simulink model "test_junk"  (Simulink 6.2)
settings: Solver=ode45  StartTime=0.0  StopTime=10.0  RelTol=1e-3
libraries: xbsIndex_r3 x670
(part 3 of 5)

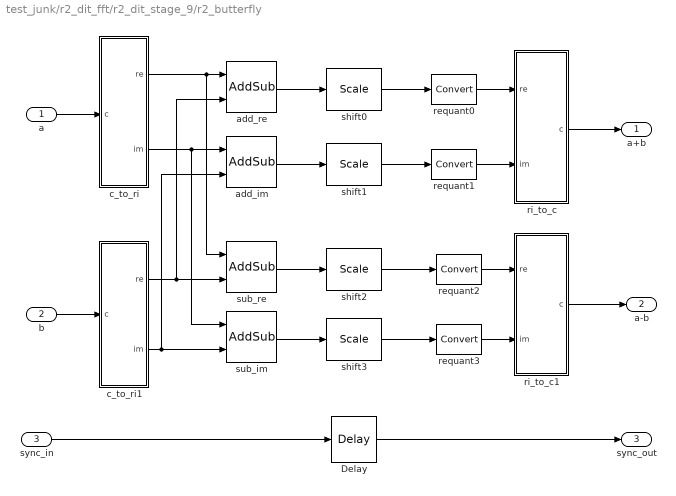
== system test_junk/r2_dit_fft/r2_dit_stage_9/r2_butterfly ==
  a : Inport  Port=1  LatchInput=off
  b : Inport  Port=2  LatchInput=off
  sync_in : Inport  Port=3  LatchInput=off
  Delay : xbsIndex_r3/Delay  latency=1  reg_retiming=off  explicit_period=off  period=1  en=off  accept_only_valid=off  init_zero=on  dbl_ovrd=off  show_param=off
      settings: xl_area=[0, 0, 0, 0, 0, 0, 0]
  add_im : xbsIndex_r3/AddSub  mode=Addition  precision=Full  arith_type=Unsigned  n_bits=8  bin_pt=2  quantization=Truncate  overflow=Wrap  latency=1  explicit_period=off  period=1  use_carryin=off  use_carryout=off  en=off  dbl_ovrd=off  show_param=on  use_core=on  pipeline=on  use_rpm=on  gen_core=off
      settings: xl_area=[0, 0, 0, 0, 0, 0, 0]
  add_re : xbsIndex_r3/AddSub  mode=Addition  precision=Full  arith_type=Unsigned  n_bits=8  bin_pt=2  quantization=Truncate  overflow=Wrap  latency=1  explicit_period=off  period=1  use_carryin=off  use_carryout=off  en=off  dbl_ovrd=off  show_param=on  use_core=on  pipeline=on  use_rpm=on  gen_core=off
      settings: xl_area=[0, 0, 0, 0, 0, 0, 0]
  c_to_ri : Subsystem
      settings: AttributesFormatString=16_0 r/i
  c_to_ri1 : Subsystem
      settings: AttributesFormatString=16_0 r/i
  requant{0..3} (4 alike) : xbsIndex_r3/Convert  arith_type="Signed  (2's comp)"  n_bits=17  bin_pt=0  quantization=Truncate  overflow=Wrap  latency=0  explicit_period=off  period=1  dbl_ovrd=off  show_param=on  inserted_by_tool=off  pipeline=on
      settings: xl_area=[0, 0, 0, 0, 0, 0, 0]
  ri_to_c : Subsystem
  ri_to_c1 : Subsystem
  shift{0..3} (4 alike) : xbsIndex_r3/Scale  scale_factor=0  explicit_period=off  period=1  dbl_ovrd=off
  sub_im : xbsIndex_r3/AddSub  mode=Subtraction  precision=Full  arith_type=Unsigned  n_bits=8  bin_pt=2  quantization=Truncate  overflow=Wrap  latency=1  explicit_period=off  period=1  use_carryin=off  use_carryout=off  en=off  dbl_ovrd=off  show_param=on  use_core=on  pipeline=on  use_rpm=on  gen_core=off
      settings: xl_area=[0, 0, 0, 0, 0, 0, 0]
  sub_re : xbsIndex_r3/AddSub  mode=Subtraction  precision=Full  arith_type=Unsigned  n_bits=8  bin_pt=2  quantization=Truncate  overflow=Wrap  latency=1  explicit_period=off  period=1  use_carryin=off  use_carryout=off  en=off  dbl_ovrd=off  show_param=on  use_core=on  pipeline=on  use_rpm=on  gen_core=off
      settings: xl_area=[0, 0, 0, 0, 0, 0, 0]
  a+b : Outport
  a-b : Outport  Port=2
  sync_out : Outport  Port=3
  wires:
  shift3/1 -> requant3/1
  sub_im/1 -> shift3/1
  shift2/1 -> requant2/1
  sub_re/1 -> shift2/1
  shift1/1 -> requant1/1
  shift0/1 -> requant0/1
  requant3/1 -> ri_to_c1/2(im)
  requant2/1 -> ri_to_c1/1(re)
  requant1/1 -> ri_to_c/2(im)
  requant0/1 -> ri_to_c/1(re)
  Delay/1 -> sync_out/1
  sync_in/1 -> Delay/1
  ri_to_c1/1(c) -> a-b/1
  ri_to_c/1(c) -> a+b/1
  add_im/1 -> shift1/1
  add_re/1 -> shift0/1
  a/1 -> c_to_ri/1(c)
  c_to_ri/2(im) -> sub_im/1, add_im/1
  c_to_ri/1(re) -> sub_re/1, add_re/1
  c_to_ri1/2(im) -> add_im/2, sub_im/2
  c_to_ri1/1(re) -> add_re/2, sub_re/2
  b/1 -> c_to_ri1/1(c)

== system test_junk/r2_dit_fft/r2_dit_stage_9/r2_twiddle ==
  a_in : Inport  Port=1  LatchInput=off
  b : Inport  Port=2  LatchInput=off
  sync_in : Inport  Port=3  LatchInput=off
  Delay1 : xbsIndex_r3/Delay  latency=1  reg_retiming=off  explicit_period=off  period=1  en=off  accept_only_valid=off  init_zero=on  dbl_ovrd=off  show_param=off
      settings: xl_area=[0, 0, 0, 0, 0, 0, 0]
  Delay2 : xbsIndex_r3/Delay  latency=1  reg_retiming=off  explicit_period=off  period=1  en=off  accept_only_valid=off  init_zero=on  dbl_ovrd=off  show_param=off
      settings: xl_area=[0, 0, 0, 0, 0, 0, 0]
  Delay3 : xbsIndex_r3/Delay  latency=1  reg_retiming=off  explicit_period=off  period=1  en=off  accept_only_valid=off  init_zero=on  dbl_ovrd=off  show_param=off
      settings: xl_area=[0, 0, 0, 0, 0, 0, 0]
  cmpy1 : Subsystem
      settings: AttributesFormatString=|
      | 16_15 * 9_7 ==> 16_15
      | round even, wrap
      | 3 mults
  twiddle_gen1 : Subsystem
      settings: AttributesFormatString=|
      | depth 256
      | twiddle bram
  a_out : Outport
  bw : Outport  Port=2
  sync_out : Outport  Port=3
  wires:
  Delay3/1 -> cmpy1/4(sync_in)
  cmpy1/3(sync_out) -> sync_out/1
  twiddle_gen1/1(w) -> cmpy1/3(w)
  cmpy1/2(bw) -> bw/1
  Delay1/1 -> cmpy1/2(b)
  cmpy1/1(a_out) -> a_out/1
  Delay2/1 -> cmpy1/1(a_in)
  a_in/1 -> Delay2/1
  b/1 -> Delay1/1
  sync_in/1 -> Delay3/1, twiddle_gen1/1(sync_in)

== system test_junk/r2_dit_fft/r2_dit_stage_1/biplex_commutator/delay_b ==
  in : Inport  Port=1  LatchInput=off
  Constant : xbsIndex_r3/Constant  const=1  equ=P=C  arith_type=Boolean  n_bits=1  bin_pt=0  opselect=C  inp2=PCIN>>17  opr=+  inp1=P  carry=CIN  iostate=0  explicit_period=on  period=1  dbl_ovrd=off
  Counter : xbsIndex_r3/Counter  cnt_type=Count Limited  n_bits=9  bin_pt=0  arith_type=Unsigned  start_count=0  cnt_to=510  cnt_by_val=1  operation=Up  explicit_period=off  period=1  load_pin=off  rst=off  en=off  dbl_ovrd=off  show_param=off  use_rpm=on  gen_core=off
      settings: xl_area=[0, 0, 0, 0, 0, 0, 0]
  bram : xbsIndex_r3/Single Port RAM  depth=512  initVector=0  write_mode=Read Before Write  latency=1  init_zero=on  explicit_period=off  period=1  rst=off  init_reg=0  en=off  dbl_ovrd=off  show_param=off  distributed_mem=off  use_rpm=off  gen_core=off
      settings: xl_area=[0, 0, 0, 0, 0, 0, 0]
  out : Outport
  wires:
  Constant/1 -> bram/3
  in/1 -> bram/2
  bram/1 -> out/1
  Counter/1 -> bram/1

== system test_junk/r2_dit_fft/r2_dit_stage_1/biplex_commutator/delay_lo ==
  in : Inport  Port=1  LatchInput=off
  Constant : xbsIndex_r3/Constant  const=1  equ=P=C  arith_type=Boolean  n_bits=1  bin_pt=0  opselect=C  inp2=PCIN>>17  opr=+  inp1=P  carry=CIN  iostate=0  explicit_period=on  period=1  dbl_ovrd=off
  Counter : xbsIndex_r3/Counter  cnt_type=Count Limited  n_bits=9  bin_pt=0  arith_type=Unsigned  start_count=0  cnt_to=510  cnt_by_val=1  operation=Up  explicit_period=off  period=1  load_pin=off  rst=off  en=off  dbl_ovrd=off  show_param=off  use_rpm=on  gen_core=off
      settings: xl_area=[0, 0, 0, 0, 0, 0, 0]
  bram : xbsIndex_r3/Single Port RAM  depth=512  initVector=0  write_mode=Read Before Write  latency=1  init_zero=on  explicit_period=off  period=1  rst=off  init_reg=0  en=off  dbl_ovrd=off  show_param=off  distributed_mem=off  use_rpm=off  gen_core=off
      settings: xl_area=[0, 0, 0, 0, 0, 0, 0]
  out : Outport
  wires:
  Constant/1 -> bram/3
  in/1 -> bram/2
  bram/1 -> out/1
  Counter/1 -> bram/1

== system test_junk/r2_dit_fft/r2_dit_stage_1/r2_butterfly/c_to_ri ==
  c : Inport  Port=1  LatchInput=off
  force_im : xbsIndex_r3/Reinterpret  force_arith_type=on  arith_type="Signed  (2's comp)"  force_bin_pt=on  bin_pt=0  force_valid=on
  force_re : xbsIndex_r3/Reinterpret  force_arith_type=on  arith_type="Signed  (2's comp)"  force_bin_pt=on  bin_pt=0  force_valid=on
  slice_im : xbsIndex_r3/Slice  mode=Lower Bit Location + Width  nbits=8  bit1=0  base1=MSB of Input  bit0=0  base0=LSB of Input  boolean_output=off  explicit_period=off  period=1  dbl_ovrd=off
  slice_re : xbsIndex_r3/Slice  mode=Upper Bit Location + Width  nbits=8  bit1=0  base1=MSB of Input  bit0=0  base0=LSB of Input  boolean_output=off  explicit_period=off  period=1  dbl_ovrd=off
  re : Outport
  im : Outport  Port=2
  wires:
  slice_re/1 -> force_re/1
  slice_im/1 -> force_im/1
  force_re/1 -> re/1
  force_im/1 -> im/1
  c/1 -> slice_re/1, slice_im/1

== system test_junk/r2_dit_fft/r2_dit_stage_1/r2_butterfly/c_to_ri1 ==
  c : Inport  Port=1  LatchInput=off
  force_im : xbsIndex_r3/Reinterpret  force_arith_type=on  arith_type="Signed  (2's comp)"  force_bin_pt=on  bin_pt=0  force_valid=on
  force_re : xbsIndex_r3/Reinterpret  force_arith_type=on  arith_type="Signed  (2's comp)"  force_bin_pt=on  bin_pt=0  force_valid=on
  slice_im : xbsIndex_r3/Slice  mode=Lower Bit Location + Width  nbits=8  bit1=0  base1=MSB of Input  bit0=0  base0=LSB of Input  boolean_output=off  explicit_period=off  period=1  dbl_ovrd=off
  slice_re : xbsIndex_r3/Slice  mode=Upper Bit Location + Width  nbits=8  bit1=0  base1=MSB of Input  bit0=0  base0=LSB of Input  boolean_output=off  explicit_period=off  period=1  dbl_ovrd=off
  re : Outport
  im : Outport  Port=2
  wires:
  slice_re/1 -> force_re/1
  slice_im/1 -> force_im/1
  force_re/1 -> re/1
  force_im/1 -> im/1
  c/1 -> slice_re/1, slice_im/1

== system test_junk/r2_dit_fft/r2_dit_stage_1/r2_butterfly/ri_to_c ==
  re : Inport  Port=1  LatchInput=off
  im : Inport  Port=2  LatchInput=off
  concat : xbsIndex_r3/Concat  num_inputs=2  explicit_period=off  period=1  dbl_ovrd=off
  force_im : xbsIndex_r3/Reinterpret  force_arith_type=on  arith_type=Unsigned  force_bin_pt=on  bin_pt=0  force_valid=on
  force_re : xbsIndex_r3/Reinterpret  force_arith_type=on  arith_type=Unsigned  force_bin_pt=on  bin_pt=0  force_valid=on
  c : Outport
  wires:
  force_re/1 -> concat/1
  force_im/1 -> concat/2
  re/1 -> force_re/1
  concat/1 -> c/1
  im/1 -> force_im/1

== system test_junk/r2_dit_fft/r2_dit_stage_1/r2_butterfly/ri_to_c1 ==
  re : Inport  Port=1  LatchInput=off
  im : Inport  Port=2  LatchInput=off
  concat : xbsIndex_r3/Concat  num_inputs=2  explicit_period=off  period=1  dbl_ovrd=off
  force_im : xbsIndex_r3/Reinterpret  force_arith_type=on  arith_type=Unsigned  force_bin_pt=on  bin_pt=0  force_valid=on
  force_re : xbsIndex_r3/Reinterpret  force_arith_type=on  arith_type=Unsigned  force_bin_pt=on  bin_pt=0  force_valid=on
  c : Outport
  wires:
  force_re/1 -> concat/1
  force_im/1 -> concat/2
  re/1 -> force_re/1
  concat/1 -> c/1
  im/1 -> force_im/1

== system test_junk/r2_dit_fft/r2_dit_stage_10/biplex_commutator/delay_b ==
  in : Inport  Port=1  LatchInput=off
  slr : xbsIndex_r3/Delay  latency=1  reg_retiming=off  explicit_period=off  period=1  en=off  accept_only_valid=off  init_zero=on  dbl_ovrd=off  show_param=off
      settings: xl_area=[0, 0, 0, 0, 0, 0, 0]
  out : Outport
  wires:
  slr/1 -> out/1
  in/1 -> slr/1

== system test_junk/r2_dit_fft/r2_dit_stage_10/biplex_commutator/delay_lo ==
  in : Inport  Port=1  LatchInput=off
  slr : xbsIndex_r3/Delay  latency=1  reg_retiming=off  explicit_period=off  period=1  en=off  accept_only_valid=off  init_zero=on  dbl_ovrd=off  show_param=off
      settings: xl_area=[0, 0, 0, 0, 0, 0, 0]
  out : Outport
  wires:
  slr/1 -> out/1
  in/1 -> slr/1

== system test_junk/r2_dit_fft/r2_dit_stage_10/r2_butterfly/c_to_ri ==
  c : Inport  Port=1  LatchInput=off
  force_im : xbsIndex_r3/Reinterpret  force_arith_type=on  arith_type="Signed  (2's comp)"  force_bin_pt=on  bin_pt=0  force_valid=on
  force_re : xbsIndex_r3/Reinterpret  force_arith_type=on  arith_type="Signed  (2's comp)"  force_bin_pt=on  bin_pt=0  force_valid=on
  slice_im : xbsIndex_r3/Slice  mode=Lower Bit Location + Width  nbits=17  bit1=0  base1=MSB of Input  bit0=0  base0=LSB of Input  boolean_output=off  explicit_period=off  period=1  dbl_ovrd=off
  slice_re : xbsIndex_r3/Slice  mode=Upper Bit Location + Width  nbits=17  bit1=0  base1=MSB of Input  bit0=0  base0=LSB of Input  boolean_output=off  explicit_period=off  period=1  dbl_ovrd=off
  re : Outport
  im : Outport  Port=2
  wires:
  slice_re/1 -> force_re/1
  slice_im/1 -> force_im/1
  force_re/1 -> re/1
  force_im/1 -> im/1
  c/1 -> slice_re/1, slice_im/1

== system test_junk/r2_dit_fft/r2_dit_stage_10/r2_butterfly/c_to_ri1 ==
  c : Inport  Port=1  LatchInput=off
  force_im : xbsIndex_r3/Reinterpret  force_arith_type=on  arith_type="Signed  (2's comp)"  force_bin_pt=on  bin_pt=0  force_valid=on
  force_re : xbsIndex_r3/Reinterpret  force_arith_type=on  arith_type="Signed  (2's comp)"  force_bin_pt=on  bin_pt=0  force_valid=on
  slice_im : xbsIndex_r3/Slice  mode=Lower Bit Location + Width  nbits=17  bit1=0  base1=MSB of Input  bit0=0  base0=LSB of Input  boolean_output=off  explicit_period=off  period=1  dbl_ovrd=off
  slice_re : xbsIndex_r3/Slice  mode=Upper Bit Location + Width  nbits=17  bit1=0  base1=MSB of Input  bit0=0  base0=LSB of Input  boolean_output=off  explicit_period=off  period=1  dbl_ovrd=off
  re : Outport
  im : Outport  Port=2
  wires:
  slice_re/1 -> force_re/1
  slice_im/1 -> force_im/1
  force_re/1 -> re/1
  force_im/1 -> im/1
  c/1 -> slice_re/1, slice_im/1

== system test_junk/r2_dit_fft/r2_dit_stage_10/r2_butterfly/ri_to_c ==
  re : Inport  Port=1  LatchInput=off
  im : Inport  Port=2  LatchInput=off
  concat : xbsIndex_r3/Concat  num_inputs=2  explicit_period=off  period=1  dbl_ovrd=off
  force_im : xbsIndex_r3/Reinterpret  force_arith_type=on  arith_type=Unsigned  force_bin_pt=on  bin_pt=0  force_valid=on
  force_re : xbsIndex_r3/Reinterpret  force_arith_type=on  arith_type=Unsigned  force_bin_pt=on  bin_pt=0  force_valid=on
  c : Outport
  wires:
  force_re/1 -> concat/1
  force_im/1 -> concat/2
  re/1 -> force_re/1
  concat/1 -> c/1
  im/1 -> force_im/1

== system test_junk/r2_dit_fft/r2_dit_stage_10/r2_butterfly/ri_to_c1 ==
  re : Inport  Port=1  LatchInput=off
  im : Inport  Port=2  LatchInput=off
  concat : xbsIndex_r3/Concat  num_inputs=2  explicit_period=off  period=1  dbl_ovrd=off
  force_im : xbsIndex_r3/Reinterpret  force_arith_type=on  arith_type=Unsigned  force_bin_pt=on  bin_pt=0  force_valid=on
  force_re : xbsIndex_r3/Reinterpret  force_arith_type=on  arith_type=Unsigned  force_bin_pt=on  bin_pt=0  force_valid=on
  c : Outport
  wires:
  force_re/1 -> concat/1
  force_im/1 -> concat/2
  re/1 -> force_re/1
  concat/1 -> c/1
  im/1 -> force_im/1

== system test_junk/r2_dit_fft/r2_dit_stage_10/r2_twiddle/cmpy1 ==
  a_in : Inport  Port=1  LatchInput=off
  b : Inport  Port=2  LatchInput=off
  w : Inport  Port=3  LatchInput=off
  sync_in : Inport  Port=4  LatchInput=off
  Delay : xbsIndex_r3/Delay  latency=8  reg_retiming=off  explicit_period=off  period=1  en=off  accept_only_valid=off  init_zero=on  dbl_ovrd=off  show_param=off
      settings: xl_area=[1 1 0 1 0 0 0]
  Delay1 : xbsIndex_r3/Delay  latency=8  reg_retiming=off  explicit_period=off  period=1  en=off  accept_only_valid=off  init_zero=on  dbl_ovrd=off  show_param=off
      settings: xl_area=[17 34 0 34 0 0 0]
  br_add_bi : xbsIndex_r3/AddSub  mode=Addition  precision=Full  arith_type=Unsigned  n_bits=8  bin_pt=2  quantization=Truncate  overflow=Wrap  latency=1  explicit_period=off  period=1  use_carryin=off  use_carryout=off  en=off  dbl_ovrd=off  show_param=on  use_core=on  pipeline=on  use_rpm=on  gen_core=off
      settings: xl_area=[9 18 0 18 0 0 0]
  c_to_ri : Subsystem
      settings: AttributesFormatString=17_16 r/i
  c_to_ri1 : Subsystem
      settings: AttributesFormatString=9_7 r/i
  convert_im : xbsIndex_r3/Convert  arith_type="Signed  (2's comp)"  n_bits=17  bin_pt=16  quantization="Round  (unbiased: Even Values)"  overflow=Wrap  latency=3  explicit_period=off  period=1  dbl_ovrd=off  show_param=on  inserted_by_tool=off  pipeline=on
      settings: xl_area=[0, 0, 0, 0, 0, 0, 0]
  convert_re : xbsIndex_r3/Convert  arith_type="Signed  (2's comp)"  n_bits=17  bin_pt=16  quantization="Round  (unbiased: Even Values)"  overflow=Wrap  latency=3  explicit_period=off  period=1  dbl_ovrd=off  show_param=on  inserted_by_tool=off  pipeline=on
      settings: xl_area=[0, 0, 0, 0, 0, 0, 0]
  imim : xbsIndex_r3/Mult  precision=User Defined  arith_type="Signed  (2's comp)"  n_bits=24  bin_pt=23  quantization=Truncate  overflow=Wrap  latency=3  explicit_period=off  period=1  en=off  dbl_ovrd=off  show_param=on  mult_type=Parallel  oversample=2  use_embedded=on  pipeline=on  use_rpm=on  placement_style=Rectangular Shape  gen_core=off
      settings: xl_area=[26 52 0 26 0 1 0]
  rere : xbsIndex_r3/Mult  precision=User Defined  arith_type="Signed  (2's comp)"  n_bits=24  bin_pt=23  quantization=Truncate  overflow=Wrap  latency=3  explicit_period=off  period=1  en=off  dbl_ovrd=off  show_param=on  mult_type=Parallel  oversample=2  use_embedded=on  pipeline=on  use_rpm=on  placement_style=Rectangular Shape  gen_core=off
      settings: xl_area=[26 52 0 26 0 1 0]
  ri_to_c : Subsystem
  rr_add_ii : xbsIndex_r3/AddSub  mode=Addition  precision=User Defined  arith_type="Signed  (2's comp)"  n_bits=24  bin_pt=23  quantization=Truncate  overflow=Wrap  latency=1  explicit_period=off  period=1  use_carryin=off  use_carryout=off  en=off  dbl_ovrd=off  show_param=on  use_core=on  pipeline=on  use_rpm=on  gen_core=off
      settings: xl_area=[14 27 0 27 0 0 0]
  rr_sub_ii : xbsIndex_r3/AddSub  mode=Subtraction  precision=User Defined  arith_type="Signed  (2's comp)"  n_bits=24  bin_pt=23  quantization=Truncate  overflow=Wrap  latency=2  explicit_period=off  period=1  use_carryin=off  use_carryout=off  en=off  dbl_ovrd=off  show_param=on  use_core=on  pipeline=on  use_rpm=on  gen_core=off
      settings: xl_area=[44 44 0 69 0 0 0]
  ss_sub_rrii : xbsIndex_r3/AddSub  mode=Subtraction  precision=User Defined  arith_type="Signed  (2's comp)"  n_bits=24  bin_pt=23  quantization=Truncate  overflow=Wrap  latency=1  explicit_period=off  period=1  use_carryin=off  use_carryout=off  en=off  dbl_ovrd=off  show_param=on  use_core=on  pipeline=on  use_rpm=on  gen_core=off
      settings: xl_area=[46 29 0 90 0 0 0]
  sumsum : xbsIndex_r3/Mult  precision=User Defined  arith_type="Signed  (2's comp)"  n_bits=24  bin_pt=23  quantization=Truncate  overflow=Wrap  latency=3  explicit_period=off  period=1  en=off  dbl_ovrd=off  show_param=on  mult_type=Parallel  oversample=2  use_embedded=on  pipeline=on  use_rpm=on  placement_style=Rectangular Shape  gen_core=off
      settings: xl_area=[28 56 0 28 0 1 0]
  wr_add_wi : xbsIndex_r3/AddSub  mode=Addition  precision=Full  arith_type=Unsigned  n_bits=8  bin_pt=2  quantization=Truncate  overflow=Wrap  latency=1  explicit_period=off  period=1  use_carryin=off  use_carryout=off  en=off  dbl_ovrd=off  show_param=on  use_core=on  pipeline=on  use_rpm=on  gen_core=off
      settings: xl_area=[5 10 0 10 0 0 0]
  a_out : Outport
  bw : Outport  Port=2
  sync_out : Outport  Port=3
  wires:
  convert_im/1 -> ri_to_c/2(im)
  convert_re/1 -> ri_to_c/1(re)
  Delay1/1 -> a_out/1
  a_in/1 -> Delay1/1
  c_to_ri/2(im) -> imim/1, br_add_bi/2
  c_to_ri1/1(re) -> wr_add_wi/1, rere/2
  c_to_ri1/2(im) -> wr_add_wi/2, imim/2
  c_to_ri/1(re) -> rere/1, br_add_bi/1
  Delay/1 -> sync_out/1
  sync_in/1 -> Delay/1
  sumsum/1 -> ss_sub_rrii/1
  ri_to_c/1(c) -> bw/1
  wr_add_wi/1 -> sumsum/2
  br_add_bi/1 -> sumsum/1
  imim/1 -> rr_add_ii/1, rr_sub_ii/2
  rere/1 -> rr_sub_ii/1, rr_add_ii/2
  w/1 -> c_to_ri1/1(c)
  b/1 -> c_to_ri/1(c)
  rr_add_ii/1 -> ss_sub_rrii/2
  rr_sub_ii/1 -> convert_re/1
  ss_sub_rrii/1 -> convert_im/1

== system test_junk/r2_dit_fft/r2_dit_stage_10/r2_twiddle/twiddle_gen1 ==
  sync_in : Inport  Port=1  LatchInput=off
  Counter : xbsIndex_r3/Counter  cnt_type=Free Running  n_bits=9  bin_pt=0  arith_type=Unsigned  start_count=0  cnt_to=Inf  cnt_by_val=1  operation=Up  explicit_period=off  period=1  load_pin=off  rst=on  en=off  dbl_ovrd=off  show_param=off  use_rpm=on  gen_core=off
      settings: xl_area=[0, 0, 0, 0, 0, 0, 0]
  addr_sel : xbsIndex_r3/Slice  mode=Upper Bit Location + Width  nbits=9  bit1=0  base1=MSB of Input  bit0=-1  base0=MSB of Input  boolean_output=off  explicit_period=off  period=1  dbl_ovrd=off
  mem_c : xbsIndex_r3/ROM  depth=512  initVector=[65536;384;47013;215973;60879;237450;25482;202191;64999;249730;36758;208313;54713;226198;13186;198119;65523;255873;41885;211887;58308;231823;19334;200155;62939;243590;31119;204740;51119;221085;7041;197619;66042;259456;44449;213930;59849;234380;22407;200661;63969;246660;34194;206270;53172;223641;10113;197613;65517;252801;39321;209844;56766;228754;16260;199137;62421;240519;28556;203209;49066;218529;3456;197114;66045;260992;45475;214952;60364;235915;23945;201682;64484;248195;35220;207292;54198;224663;11650;198122;65520;254337;40859;210865;57281;230289;17797;199646;62936;242054;30094;204230;50092;219551;4992;197111;66039;257920;43423;212908;58822;232846;20870;200152;63454;245125;32657;205761;52145;222107;8577;197616;65002;251266;38295;208822;55740;227732;14723;198628;61394;238985;27019;202700;48040;217507;1920;197117;66046;261504;45988;215463;60878;236938;24969;201680;64485;248707;36245;207802;54712;225686;12162;198121;65522;255361;41372;211376;57794;230800;18821;199644;62937;242566;30606;204229;50606;220574;6016;197109;66040;258432;43936;213419;59336;233869;21895;200662;63967;245636;33169;205760;52658;222618;9089;197615;65004;252290;38808;209333;56253;228243;15747;198626;61907;239496;27532;203211;48553;218018;2944;197115;66043;259968;44962;214441;59851;235404;23432;201171;64482;247171;34707;206781;53685;224152;10626;198124;65519;253825;40346;210354;57280;229777;17284;199135;62422;241031;29069;203720;49579;219040;4480;197112;66037;256896;42398;212398;58821;232334;20358;200153;63452;244101;32144;205250;51632;221596;7553;197618;65001;250754;37270;208312;55226;226709;14211;198629;61392;237961;25994;202190;47527;216996;1408;197118;66047;262016;46501;215974;60878;236938;24969;201680;64486;249219;36245;207802;54712;225686;12674;198120;65523;255873;41885;211887;58307;231311;18821;199644;62938;243078;31119;204740;50606;220574;6529;197620;66041;258944;43937;213931;59337;234381;21895;200662;63968;246148;33682;206271;52659;223130;9601;197614;65004;252290;39321;209844;56254;228755;15748;199138;61908;240008;28044;203210;48553;218018;2944;197115;66044;260480;45475;214952;60363;235403;23432;201171;64483;247683;35219;206780;53686;224664;11138;198123;65520;254337;40347;210866;57280;229777;17284;199135;62423;241543;29581;203719;49580;219552;4992;197111;66038;257408;42911;212909;58822;232846;20358;200153;63453;244613;32144;205250;51633;222108;8065;197617;65001;250754;37783;208823;55739;227220;14211;198629;61393;238473;26507;202701;47527;216996;1408;197118;66046;261504;45988;215463;60365;236427;24457;201681;64485;248707;35732;207291;54199;225175;12162;198121;65521;254849;40860;211377;57794;230800;18309;199645;62937;242566;30094;204230;50093;220063;5504;197110;66039;257920;43424;213420;59335;233357;21383;200663;63967;245636;33169;205760;52146;222619;8577;197616;65003;251778;38296;209334;56252;227731;15235;198627;61907;239496;27531;202699;48040;217507;2432;197116;66043;259968;44962;214441;59850;234892;22920;201172;63970;247172;34195;206782;53172;223641;10626;198124;65518;253313;39834;210355;56767;229266;16772;199136;62422;241031;28557;203721;49067;219041;3968;197113;65524;256385;42398;212398;58308;231823;19846;200154;63452;244101;31631;204739;51119;221085;7041;197619;65000;250242;37270;208312;55226;226709;13699;198630;61392;237961;25994;202190;47014;216485;896;197119]  arith_type=Unsigned  n_bits=18  bin_pt=0  latency=1  init_zero=on  explicit_period=off  period=1  rst=off  init_reg=0  en=off  dbl_ovrd=off  show_param=on  distributed_mem=off  use_rpm=on  gen_core=off
      settings: AttributesFormatString=depth = %<depth>\ndist_mem = %<distributed_mem>  xl_area=[0, 0, 0, 0, 0, 0, 0]
  w : Outport
  wires:
  mem_c/1 -> w/1
  addr_sel/1 -> mem_c/1
  Counter/1 -> addr_sel/1
  sync_in/1 -> Counter/1

== system test_junk/r2_dit_fft/r2_dit_stage_2/biplex_commutator/delay_b ==
  in : Inport  Port=1  LatchInput=off
  Constant : xbsIndex_r3/Constant  const=1  equ=P=C  arith_type=Boolean  n_bits=1  bin_pt=0  opselect=C  inp2=PCIN>>17  opr=+  inp1=P  carry=CIN  iostate=0  explicit_period=on  period=1  dbl_ovrd=off
  Counter : xbsIndex_r3/Counter  cnt_type=Count Limited  n_bits=8  bin_pt=0  arith_type=Unsigned  start_count=0  cnt_to=254  cnt_by_val=1  operation=Up  explicit_period=off  period=1  load_pin=off  rst=off  en=off  dbl_ovrd=off  show_param=off  use_rpm=on  gen_core=off
      settings: xl_area=[0, 0, 0, 0, 0, 0, 0]
  bram : xbsIndex_r3/Single Port RAM  depth=256  initVector=0  write_mode=Read Before Write  latency=1  init_zero=on  explicit_period=off  period=1  rst=off  init_reg=0  en=off  dbl_ovrd=off  show_param=off  distributed_mem=off  use_rpm=off  gen_core=off
      settings: xl_area=[0, 0, 0, 0, 0, 0, 0]
  out : Outport
  wires:
  Constant/1 -> bram/3
  in/1 -> bram/2
  bram/1 -> out/1
  Counter/1 -> bram/1

== system test_junk/r2_dit_fft/r2_dit_stage_2/biplex_commutator/delay_lo ==
  in : Inport  Port=1  LatchInput=off
  Constant : xbsIndex_r3/Constant  const=1  equ=P=C  arith_type=Boolean  n_bits=1  bin_pt=0  opselect=C  inp2=PCIN>>17  opr=+  inp1=P  carry=CIN  iostate=0  explicit_period=on  period=1  dbl_ovrd=off
  Counter : xbsIndex_r3/Counter  cnt_type=Count Limited  n_bits=8  bin_pt=0  arith_type=Unsigned  start_count=0  cnt_to=254  cnt_by_val=1  operation=Up  explicit_period=off  period=1  load_pin=off  rst=off  en=off  dbl_ovrd=off  show_param=off  use_rpm=on  gen_core=off
      settings: xl_area=[0, 0, 0, 0, 0, 0, 0]
  bram : xbsIndex_r3/Single Port RAM  depth=256  initVector=0  write_mode=Read Before Write  latency=1  init_zero=on  explicit_period=off  period=1  rst=off  init_reg=0  en=off  dbl_ovrd=off  show_param=off  distributed_mem=off  use_rpm=off  gen_core=off
      settings: xl_area=[0, 0, 0, 0, 0, 0, 0]
  out : Outport
  wires:
  Constant/1 -> bram/3
  in/1 -> bram/2
  bram/1 -> out/1
  Counter/1 -> bram/1

== system test_junk/r2_dit_fft/r2_dit_stage_2/r2_butterfly/c_to_ri ==
  c : Inport  Port=1  LatchInput=off
  force_im : xbsIndex_r3/Reinterpret  force_arith_type=on  arith_type="Signed  (2's comp)"  force_bin_pt=on  bin_pt=0  force_valid=on
  force_re : xbsIndex_r3/Reinterpret  force_arith_type=on  arith_type="Signed  (2's comp)"  force_bin_pt=on  bin_pt=0  force_valid=on
  slice_im : xbsIndex_r3/Slice  mode=Lower Bit Location + Width  nbits=9  bit1=0  base1=MSB of Input  bit0=0  base0=LSB of Input  boolean_output=off  explicit_period=off  period=1  dbl_ovrd=off
  slice_re : xbsIndex_r3/Slice  mode=Upper Bit Location + Width  nbits=9  bit1=0  base1=MSB of Input  bit0=0  base0=LSB of Input  boolean_output=off  explicit_period=off  period=1  dbl_ovrd=off
  re : Outport
  im : Outport  Port=2
  wires:
  slice_re/1 -> force_re/1
  slice_im/1 -> force_im/1
  force_re/1 -> re/1
  force_im/1 -> im/1
  c/1 -> slice_re/1, slice_im/1

== system test_junk/r2_dit_fft/r2_dit_stage_2/r2_butterfly/c_to_ri1 ==
  c : Inport  Port=1  LatchInput=off
  force_im : xbsIndex_r3/Reinterpret  force_arith_type=on  arith_type="Signed  (2's comp)"  force_bin_pt=on  bin_pt=0  force_valid=on
  force_re : xbsIndex_r3/Reinterpret  force_arith_type=on  arith_type="Signed  (2's comp)"  force_bin_pt=on  bin_pt=0  force_valid=on
  slice_im : xbsIndex_r3/Slice  mode=Lower Bit Location + Width  nbits=9  bit1=0  base1=MSB of Input  bit0=0  base0=LSB of Input  boolean_output=off  explicit_period=off  period=1  dbl_ovrd=off
  slice_re : xbsIndex_r3/Slice  mode=Upper Bit Location + Width  nbits=9  bit1=0  base1=MSB of Input  bit0=0  base0=LSB of Input  boolean_output=off  explicit_period=off  period=1  dbl_ovrd=off
  re : Outport
  im : Outport  Port=2
  wires:
  slice_re/1 -> force_re/1
  slice_im/1 -> force_im/1
  force_re/1 -> re/1
  force_im/1 -> im/1
  c/1 -> slice_re/1, slice_im/1

== system test_junk/r2_dit_fft/r2_dit_stage_2/r2_butterfly/ri_to_c ==
  re : Inport  Port=1  LatchInput=off
  im : Inport  Port=2  LatchInput=off
  concat : xbsIndex_r3/Concat  num_inputs=2  explicit_period=off  period=1  dbl_ovrd=off
  force_im : xbsIndex_r3/Reinterpret  force_arith_type=on  arith_type=Unsigned  force_bin_pt=on  bin_pt=0  force_valid=on
  force_re : xbsIndex_r3/Reinterpret  force_arith_type=on  arith_type=Unsigned  force_bin_pt=on  bin_pt=0  force_valid=on
  c : Outport
  wires:
  force_re/1 -> concat/1
  force_im/1 -> concat/2
  re/1 -> force_re/1
  concat/1 -> c/1
  im/1 -> force_im/1

== system test_junk/r2_dit_fft/r2_dit_stage_2/r2_butterfly/ri_to_c1 ==
  re : Inport  Port=1  LatchInput=off
  im : Inport  Port=2  LatchInput=off
  concat : xbsIndex_r3/Concat  num_inputs=2  explicit_period=off  period=1  dbl_ovrd=off
  force_im : xbsIndex_r3/Reinterpret  force_arith_type=on  arith_type=Unsigned  force_bin_pt=on  bin_pt=0  force_valid=on
  force_re : xbsIndex_r3/Reinterpret  force_arith_type=on  arith_type=Unsigned  force_bin_pt=on  bin_pt=0  force_valid=on
  c : Outport
  wires:
  force_re/1 -> concat/1
  force_im/1 -> concat/2
  re/1 -> force_re/1
  concat/1 -> c/1
  im/1 -> force_im/1

== system test_junk/r2_dit_fft/r2_dit_stage_3/biplex_commutator/delay_b ==
  in : Inport  Port=1  LatchInput=off
  c_to_ri : Subsystem
      settings: AttributesFormatString=10_0 r/i
  delay_im : Subsystem
      settings: AttributesFormatString=bram depth = 128
  delay_re : Subsystem
      settings: AttributesFormatString=bram depth = 128
  ri_to_c : Subsystem
  out : Outport
  wires:
  delay_im/1(out) -> ri_to_c/2(im)
  c_to_ri/2(im) -> delay_im/1(in)
  ri_to_c/1(c) -> out/1
  delay_re/1(out) -> ri_to_c/1(re)
  c_to_ri/1(re) -> delay_re/1(in)
  in/1 -> c_to_ri/1(c)

== system test_junk/r2_dit_fft/r2_dit_stage_3/biplex_commutator/delay_lo ==
  in : Inport  Port=1  LatchInput=off
  c_to_ri : Subsystem
      settings: AttributesFormatString=10_0 r/i
  delay_im : Subsystem
      settings: AttributesFormatString=bram depth = 128
  delay_re : Subsystem
      settings: AttributesFormatString=bram depth = 128
  ri_to_c : Subsystem
  out : Outport
  wires:
  delay_im/1(out) -> ri_to_c/2(im)
  c_to_ri/2(im) -> delay_im/1(in)
  ri_to_c/1(c) -> out/1
  delay_re/1(out) -> ri_to_c/1(re)
  c_to_ri/1(re) -> delay_re/1(in)
  in/1 -> c_to_ri/1(c)

== system test_junk/r2_dit_fft/r2_dit_stage_3/r2_butterfly/c_to_ri ==
  c : Inport  Port=1  LatchInput=off
  force_im : xbsIndex_r3/Reinterpret  force_arith_type=on  arith_type="Signed  (2's comp)"  force_bin_pt=on  bin_pt=0  force_valid=on
  force_re : xbsIndex_r3/Reinterpret  force_arith_type=on  arith_type="Signed  (2's comp)"  force_bin_pt=on  bin_pt=0  force_valid=on
  slice_im : xbsIndex_r3/Slice  mode=Lower Bit Location + Width  nbits=10  bit1=0  base1=MSB of Input  bit0=0  base0=LSB of Input  boolean_output=off  explicit_period=off  period=1  dbl_ovrd=off
  slice_re : xbsIndex_r3/Slice  mode=Upper Bit Location + Width  nbits=10  bit1=0  base1=MSB of Input  bit0=0  base0=LSB of Input  boolean_output=off  explicit_period=off  period=1  dbl_ovrd=off
  re : Outport
  im : Outport  Port=2
  wires:
  slice_re/1 -> force_re/1
  slice_im/1 -> force_im/1
  force_re/1 -> re/1
  force_im/1 -> im/1
  c/1 -> slice_re/1, slice_im/1

== system test_junk/r2_dit_fft/r2_dit_stage_3/r2_butterfly/c_to_ri1 ==
  c : Inport  Port=1  LatchInput=off
  force_im : xbsIndex_r3/Reinterpret  force_arith_type=on  arith_type="Signed  (2's comp)"  force_bin_pt=on  bin_pt=0  force_valid=on
  force_re : xbsIndex_r3/Reinterpret  force_arith_type=on  arith_type="Signed  (2's comp)"  force_bin_pt=on  bin_pt=0  force_valid=on
  slice_im : xbsIndex_r3/Slice  mode=Lower Bit Location + Width  nbits=10  bit1=0  base1=MSB of Input  bit0=0  base0=LSB of Input  boolean_output=off  explicit_period=off  period=1  dbl_ovrd=off
  slice_re : xbsIndex_r3/Slice  mode=Upper Bit Location + Width  nbits=10  bit1=0  base1=MSB of Input  bit0=0  base0=LSB of Input  boolean_output=off  explicit_period=off  period=1  dbl_ovrd=off
  re : Outport
  im : Outport  Port=2
  wires:
  slice_re/1 -> force_re/1
  slice_im/1 -> force_im/1
  force_re/1 -> re/1
  force_im/1 -> im/1
  c/1 -> slice_re/1, slice_im/1

== system test_junk/r2_dit_fft/r2_dit_stage_3/r2_butterfly/ri_to_c ==
  re : Inport  Port=1  LatchInput=off
  im : Inport  Port=2  LatchInput=off
  concat : xbsIndex_r3/Concat  num_inputs=2  explicit_period=off  period=1  dbl_ovrd=off
  force_im : xbsIndex_r3/Reinterpret  force_arith_type=on  arith_type=Unsigned  force_bin_pt=on  bin_pt=0  force_valid=on
  force_re : xbsIndex_r3/Reinterpret  force_arith_type=on  arith_type=Unsigned  force_bin_pt=on  bin_pt=0  force_valid=on
  c : Outport
  wires:
  force_re/1 -> concat/1
  force_im/1 -> concat/2
  re/1 -> force_re/1
  concat/1 -> c/1
  im/1 -> force_im/1

== system test_junk/r2_dit_fft/r2_dit_stage_3/r2_butterfly/ri_to_c1 ==
  re : Inport  Port=1  LatchInput=off
  im : Inport  Port=2  LatchInput=off
  concat : xbsIndex_r3/Concat  num_inputs=2  explicit_period=off  period=1  dbl_ovrd=off
  force_im : xbsIndex_r3/Reinterpret  force_arith_type=on  arith_type=Unsigned  force_bin_pt=on  bin_pt=0  force_valid=on
  force_re : xbsIndex_r3/Reinterpret  force_arith_type=on  arith_type=Unsigned  force_bin_pt=on  bin_pt=0  force_valid=on
  c : Outport
  wires:
  force_re/1 -> concat/1
  force_im/1 -> concat/2
  re/1 -> force_re/1
  concat/1 -> c/1
  im/1 -> force_im/1

== system test_junk/r2_dit_fft/r2_dit_stage_3/r2_twiddle/cmpy1 ==
  a_in : Inport  Port=1  LatchInput=off
  b : Inport  Port=2  LatchInput=off
  w : Inport  Port=3  LatchInput=off
  sync_in : Inport  Port=4  LatchInput=off
  Delay : xbsIndex_r3/Delay  latency=8  reg_retiming=off  explicit_period=off  period=1  en=off  accept_only_valid=off  init_zero=on  dbl_ovrd=off  show_param=off
      settings: xl_area=[1 1 0 1 0 0 0]
  Delay1 : xbsIndex_r3/Delay  latency=8  reg_retiming=off  explicit_period=off  period=1  en=off  accept_only_valid=off  init_zero=on  dbl_ovrd=off  show_param=off
      settings: xl_area=[17 34 0 34 0 0 0]
  br_add_bi : xbsIndex_r3/AddSub  mode=Addition  precision=Full  arith_type=Unsigned  n_bits=8  bin_pt=2  quantization=Truncate  overflow=Wrap  latency=1  explicit_period=off  period=1  use_carryin=off  use_carryout=off  en=off  dbl_ovrd=off  show_param=on  use_core=on  pipeline=on  use_rpm=on  gen_core=off
      settings: xl_area=[9 18 0 18 0 0 0]
  c_to_ri : Subsystem
      settings: AttributesFormatString=10_9 r/i
  c_to_ri1 : Subsystem
      settings: AttributesFormatString=9_7 r/i
  convert_im : xbsIndex_r3/Convert  arith_type="Signed  (2's comp)"  n_bits=10  bin_pt=9  quantization="Round  (unbiased: Even Values)"  overflow=Wrap  latency=3  explicit_period=off  period=1  dbl_ovrd=off  show_param=on  inserted_by_tool=off  pipeline=on
      settings: xl_area=[0, 0, 0, 0, 0, 0, 0]
  convert_re : xbsIndex_r3/Convert  arith_type="Signed  (2's comp)"  n_bits=10  bin_pt=9  quantization="Round  (unbiased: Even Values)"  overflow=Wrap  latency=3  explicit_period=off  period=1  dbl_ovrd=off  show_param=on  inserted_by_tool=off  pipeline=on
      settings: xl_area=[0, 0, 0, 0, 0, 0, 0]
  imim : xbsIndex_r3/Mult  precision=User Defined  arith_type="Signed  (2's comp)"  n_bits=17  bin_pt=16  quantization=Truncate  overflow=Wrap  latency=3  explicit_period=off  period=1  en=off  dbl_ovrd=off  show_param=on  mult_type=Parallel  oversample=2  use_embedded=on  pipeline=on  use_rpm=on  placement_style=Rectangular Shape  gen_core=off
      settings: xl_area=[26 52 0 26 0 1 0]
  rere : xbsIndex_r3/Mult  precision=User Defined  arith_type="Signed  (2's comp)"  n_bits=17  bin_pt=16  quantization=Truncate  overflow=Wrap  latency=3  explicit_period=off  period=1  en=off  dbl_ovrd=off  show_param=on  mult_type=Parallel  oversample=2  use_embedded=on  pipeline=on  use_rpm=on  placement_style=Rectangular Shape  gen_core=off
      settings: xl_area=[26 52 0 26 0 1 0]
  ri_to_c : Subsystem
  rr_add_ii : xbsIndex_r3/AddSub  mode=Addition  precision=User Defined  arith_type="Signed  (2's comp)"  n_bits=17  bin_pt=16  quantization=Truncate  overflow=Wrap  latency=1  explicit_period=off  period=1  use_carryin=off  use_carryout=off  en=off  dbl_ovrd=off  show_param=on  use_core=on  pipeline=on  use_rpm=on  gen_core=off
      settings: xl_area=[14 27 0 27 0 0 0]
  rr_sub_ii : xbsIndex_r3/AddSub  mode=Subtraction  precision=User Defined  arith_type="Signed  (2's comp)"  n_bits=17  bin_pt=16  quantization=Truncate  overflow=Wrap  latency=2  explicit_period=off  period=1  use_carryin=off  use_carryout=off  en=off  dbl_ovrd=off  show_param=on  use_core=on  pipeline=on  use_rpm=on  gen_core=off
      settings: xl_area=[44 44 0 69 0 0 0]
  ss_sub_rrii : xbsIndex_r3/AddSub  mode=Subtraction  precision=User Defined  arith_type="Signed  (2's comp)"  n_bits=17  bin_pt=16  quantization=Truncate  overflow=Wrap  latency=1  explicit_period=off  period=1  use_carryin=off  use_carryout=off  en=off  dbl_ovrd=off  show_param=on  use_core=on  pipeline=on  use_rpm=on  gen_core=off
      settings: xl_area=[46 29 0 90 0 0 0]
  sumsum : xbsIndex_r3/Mult  precision=User Defined  arith_type="Signed  (2's comp)"  n_bits=17  bin_pt=16  quantization=Truncate  overflow=Wrap  latency=3  explicit_period=off  period=1  en=off  dbl_ovrd=off  show_param=on  mult_type=Parallel  oversample=2  use_embedded=on  pipeline=on  use_rpm=on  placement_style=Rectangular Shape  gen_core=off
      settings: xl_area=[28 56 0 28 0 1 0]
  wr_add_wi : xbsIndex_r3/AddSub  mode=Addition  precision=Full  arith_type=Unsigned  n_bits=8  bin_pt=2  quantization=Truncate  overflow=Wrap  latency=1  explicit_period=off  period=1  use_carryin=off  use_carryout=off  en=off  dbl_ovrd=off  show_param=on  use_core=on  pipeline=on  use_rpm=on  gen_core=off
      settings: xl_area=[5 10 0 10 0 0 0]
  a_out : Outport
  bw : Outport  Port=2
  sync_out : Outport  Port=3
  wires:
  convert_im/1 -> ri_to_c/2(im)
  convert_re/1 -> ri_to_c/1(re)
  Delay1/1 -> a_out/1
  a_in/1 -> Delay1/1
  c_to_ri/2(im) -> imim/1, br_add_bi/2
  c_to_ri1/1(re) -> wr_add_wi/1, rere/2
  c_to_ri1/2(im) -> wr_add_wi/2, imim/2
  c_to_ri/1(re) -> rere/1, br_add_bi/1
  Delay/1 -> sync_out/1
  sync_in/1 -> Delay/1
  sumsum/1 -> ss_sub_rrii/1
  ri_to_c/1(c) -> bw/1
  wr_add_wi/1 -> sumsum/2
  br_add_bi/1 -> sumsum/1
  imim/1 -> rr_add_ii/1, rr_sub_ii/2
  rere/1 -> rr_sub_ii/1, rr_add_ii/2
  w/1 -> c_to_ri1/1(c)
  b/1 -> c_to_ri/1(c)
  rr_add_ii/1 -> ss_sub_rrii/2
  rr_sub_ii/1 -> convert_re/1
  ss_sub_rrii/1 -> convert_im/1

== system test_junk/r2_dit_fft/r2_dit_stage_3/r2_twiddle/twiddle_gen1 ==
  sync_in : Inport  Port=1  LatchInput=off
  Counter : xbsIndex_r3/Counter  cnt_type=Free Running  n_bits=9  bin_pt=0  arith_type=Unsigned  start_count=0  cnt_to=Inf  cnt_by_val=1  operation=Up  explicit_period=off  period=1  load_pin=off  rst=on  en=off  dbl_ovrd=off  show_param=off  use_rpm=on  gen_core=off
      settings: xl_area=[0, 0, 0, 0, 0, 0, 0]
  addr_sel : xbsIndex_r3/Slice  mode=Upper Bit Location + Width  nbits=2  bit1=0  base1=MSB of Input  bit0=-1  base0=MSB of Input  boolean_output=off  explicit_period=off  period=1  dbl_ovrd=off
  mem_c : xbsIndex_r3/ROM  depth=4  initVector=[65536;384;47013;215973]  arith_type=Unsigned  n_bits=18  bin_pt=0  latency=1  init_zero=on  explicit_period=off  period=1  rst=off  init_reg=0  en=off  dbl_ovrd=off  show_param=on  distributed_mem=on  use_rpm=on  gen_core=off
      settings: AttributesFormatString=depth = %<depth>\ndist_mem = %<distributed_mem>  xl_area=[0, 0, 0, 0, 0, 0, 0]
  w : Outport
  wires:
  mem_c/1 -> w/1
  addr_sel/1 -> mem_c/1
  Counter/1 -> addr_sel/1
  sync_in/1 -> Counter/1

== system test_junk/r2_dit_fft/r2_dit_stage_4/biplex_commutator/delay_b ==
  in : Inport  Port=1  LatchInput=off
  slr : xbsIndex_r3/Delay  latency=64  reg_retiming=off  explicit_period=off  period=1  en=off  accept_only_valid=off  init_zero=on  dbl_ovrd=off  show_param=off
      settings: xl_area=[0, 0, 0, 0, 0, 0, 0]
  out : Outport
  wires:
  slr/1 -> out/1
  in/1 -> slr/1

== system test_junk/r2_dit_fft/r2_dit_stage_4/biplex_commutator/delay_lo ==
  in : Inport  Port=1  LatchInput=off
  slr : xbsIndex_r3/Delay  latency=64  reg_retiming=off  explicit_period=off  period=1  en=off  accept_only_valid=off  init_zero=on  dbl_ovrd=off  show_param=off
      settings: xl_area=[0, 0, 0, 0, 0, 0, 0]
  out : Outport
  wires:
  slr/1 -> out/1
  in/1 -> slr/1

== system test_junk/r2_dit_fft/r2_dit_stage_4/r2_butterfly/c_to_ri ==
  c : Inport  Port=1  LatchInput=off
  force_im : xbsIndex_r3/Reinterpret  force_arith_type=on  arith_type="Signed  (2's comp)"  force_bin_pt=on  bin_pt=0  force_valid=on
  force_re : xbsIndex_r3/Reinterpret  force_arith_type=on  arith_type="Signed  (2's comp)"  force_bin_pt=on  bin_pt=0  force_valid=on
  slice_im : xbsIndex_r3/Slice  mode=Lower Bit Location + Width  nbits=11  bit1=0  base1=MSB of Input  bit0=0  base0=LSB of Input  boolean_output=off  explicit_period=off  period=1  dbl_ovrd=off
  slice_re : xbsIndex_r3/Slice  mode=Upper Bit Location + Width  nbits=11  bit1=0  base1=MSB of Input  bit0=0  base0=LSB of Input  boolean_output=off  explicit_period=off  period=1  dbl_ovrd=off
  re : Outport
  im : Outport  Port=2
  wires:
  slice_re/1 -> force_re/1
  slice_im/1 -> force_im/1
  force_re/1 -> re/1
  force_im/1 -> im/1
  c/1 -> slice_re/1, slice_im/1

== system test_junk/r2_dit_fft/r2_dit_stage_4/r2_butterfly/c_to_ri1 ==
  c : Inport  Port=1  LatchInput=off
  force_im : xbsIndex_r3/Reinterpret  force_arith_type=on  arith_type="Signed  (2's comp)"  force_bin_pt=on  bin_pt=0  force_valid=on
  force_re : xbsIndex_r3/Reinterpret  force_arith_type=on  arith_type="Signed  (2's comp)"  force_bin_pt=on  bin_pt=0  force_valid=on
  slice_im : xbsIndex_r3/Slice  mode=Lower Bit Location + Width  nbits=11  bit1=0  base1=MSB of Input  bit0=0  base0=LSB of Input  boolean_output=off  explicit_period=off  period=1  dbl_ovrd=off
  slice_re : xbsIndex_r3/Slice  mode=Upper Bit Location + Width  nbits=11  bit1=0  base1=MSB of Input  bit0=0  base0=LSB of Input  boolean_output=off  explicit_period=off  period=1  dbl_ovrd=off
  re : Outport
  im : Outport  Port=2
  wires:
  slice_re/1 -> force_re/1
  slice_im/1 -> force_im/1
  force_re/1 -> re/1
  force_im/1 -> im/1
  c/1 -> slice_re/1, slice_im/1

== system test_junk/r2_dit_fft/r2_dit_stage_4/r2_butterfly/ri_to_c ==
  re : Inport  Port=1  LatchInput=off
  im : Inport  Port=2  LatchInput=off
  concat : xbsIndex_r3/Concat  num_inputs=2  explicit_period=off  period=1  dbl_ovrd=off
  force_im : xbsIndex_r3/Reinterpret  force_arith_type=on  arith_type=Unsigned  force_bin_pt=on  bin_pt=0  force_valid=on
  force_re : xbsIndex_r3/Reinterpret  force_arith_type=on  arith_type=Unsigned  force_bin_pt=on  bin_pt=0  force_valid=on
  c : Outport
  wires:
  force_re/1 -> concat/1
  force_im/1 -> concat/2
  re/1 -> force_re/1
  concat/1 -> c/1
  im/1 -> force_im/1

== system test_junk/r2_dit_fft/r2_dit_stage_4/r2_butterfly/ri_to_c1 ==
  re : Inport  Port=1  LatchInput=off
  im : Inport  Port=2  LatchInput=off
  concat : xbsIndex_r3/Concat  num_inputs=2  explicit_period=off  period=1  dbl_ovrd=off
  force_im : xbsIndex_r3/Reinterpret  force_arith_type=on  arith_type=Unsigned  force_bin_pt=on  bin_pt=0  force_valid=on
  force_re : xbsIndex_r3/Reinterpret  force_arith_type=on  arith_type=Unsigned  force_bin_pt=on  bin_pt=0  force_valid=on
  c : Outport
  wires:
  force_re/1 -> concat/1
  force_im/1 -> concat/2
  re/1 -> force_re/1
  concat/1 -> c/1
  im/1 -> force_im/1

== system test_junk/r2_dit_fft/r2_dit_stage_4/r2_twiddle/cmpy1 ==
  a_in : Inport  Port=1  LatchInput=off
  b : Inport  Port=2  LatchInput=off
  w : Inport  Port=3  LatchInput=off
  sync_in : Inport  Port=4  LatchInput=off
  Delay : xbsIndex_r3/Delay  latency=8  reg_retiming=off  explicit_period=off  period=1  en=off  accept_only_valid=off  init_zero=on  dbl_ovrd=off  show_param=off
      settings: xl_area=[1 1 0 1 0 0 0]
  Delay1 : xbsIndex_r3/Delay  latency=8  reg_retiming=off  explicit_period=off  period=1  en=off  accept_only_valid=off  init_zero=on  dbl_ovrd=off  show_param=off
      settings: xl_area=[17 34 0 34 0 0 0]
  br_add_bi : xbsIndex_r3/AddSub  mode=Addition  precision=Full  arith_type=Unsigned  n_bits=8  bin_pt=2  quantization=Truncate  overflow=Wrap  latency=1  explicit_period=off  period=1  use_carryin=off  use_carryout=off  en=off  dbl_ovrd=off  show_param=on  use_core=on  pipeline=on  use_rpm=on  gen_core=off
      settings: xl_area=[9 18 0 18 0 0 0]
  c_to_ri : Subsystem
      settings: AttributesFormatString=11_10 r/i
  c_to_ri1 : Subsystem
      settings: AttributesFormatString=9_7 r/i
  convert_im : xbsIndex_r3/Convert  arith_type="Signed  (2's comp)"  n_bits=11  bin_pt=10  quantization="Round  (unbiased: Even Values)"  overflow=Wrap  latency=3  explicit_period=off  period=1  dbl_ovrd=off  show_param=on  inserted_by_tool=off  pipeline=on
      settings: xl_area=[0, 0, 0, 0, 0, 0, 0]
  convert_re : xbsIndex_r3/Convert  arith_type="Signed  (2's comp)"  n_bits=11  bin_pt=10  quantization="Round  (unbiased: Even Values)"  overflow=Wrap  latency=3  explicit_period=off  period=1  dbl_ovrd=off  show_param=on  inserted_by_tool=off  pipeline=on
      settings: xl_area=[0, 0, 0, 0, 0, 0, 0]
  imim : xbsIndex_r3/Mult  precision=User Defined  arith_type="Signed  (2's comp)"  n_bits=18  bin_pt=17  quantization=Truncate  overflow=Wrap  latency=3  explicit_period=off  period=1  en=off  dbl_ovrd=off  show_param=on  mult_type=Parallel  oversample=2  use_embedded=on  pipeline=on  use_rpm=on  placement_style=Rectangular Shape  gen_core=off
      settings: xl_area=[26 52 0 26 0 1 0]
  rere : xbsIndex_r3/Mult  precision=User Defined  arith_type="Signed  (2's comp)"  n_bits=18  bin_pt=17  quantization=Truncate  overflow=Wrap  latency=3  explicit_period=off  period=1  en=off  dbl_ovrd=off  show_param=on  mult_type=Parallel  oversample=2  use_embedded=on  pipeline=on  use_rpm=on  placement_style=Rectangular Shape  gen_core=off
      settings: xl_area=[26 52 0 26 0 1 0]
  ri_to_c : Subsystem
  rr_add_ii : xbsIndex_r3/AddSub  mode=Addition  precision=User Defined  arith_type="Signed  (2's comp)"  n_bits=18  bin_pt=17  quantization=Truncate  overflow=Wrap  latency=1  explicit_period=off  period=1  use_carryin=off  use_carryout=off  en=off  dbl_ovrd=off  show_param=on  use_core=on  pipeline=on  use_rpm=on  gen_core=off
      settings: xl_area=[14 27 0 27 0 0 0]
  rr_sub_ii : xbsIndex_r3/AddSub  mode=Subtraction  precision=User Defined  arith_type="Signed  (2's comp)"  n_bits=18  bin_pt=17  quantization=Truncate  overflow=Wrap  latency=2  explicit_period=off  period=1  use_carryin=off  use_carryout=off  en=off  dbl_ovrd=off  show_param=on  use_core=on  pipeline=on  use_rpm=on  gen_core=off
      settings: xl_area=[44 44 0 69 0 0 0]
  ss_sub_rrii : xbsIndex_r3/AddSub  mode=Subtraction  precision=User Defined  arith_type="Signed  (2's comp)"  n_bits=18  bin_pt=17  quantization=Truncate  overflow=Wrap  latency=1  explicit_period=off  period=1  use_carryin=off  use_carryout=off  en=off  dbl_ovrd=off  show_param=on  use_core=on  pipeline=on  use_rpm=on  gen_core=off
      settings: xl_area=[46 29 0 90 0 0 0]
  sumsum : xbsIndex_r3/Mult  precision=User Defined  arith_type="Signed  (2's comp)"  n_bits=18  bin_pt=17  quantization=Truncate  overflow=Wrap  latency=3  explicit_period=off  period=1  en=off  dbl_ovrd=off  show_param=on  mult_type=Parallel  oversample=2  use_embedded=on  pipeline=on  use_rpm=on  placement_style=Rectangular Shape  gen_core=off
      settings: xl_area=[28 56 0 28 0 1 0]
  wr_add_wi : xbsIndex_r3/AddSub  mode=Addition  precision=Full  arith_type=Unsigned  n_bits=8  bin_pt=2  quantization=Truncate  overflow=Wrap  latency=1  explicit_period=off  period=1  use_carryin=off  use_carryout=off  en=off  dbl_ovrd=off  show_param=on  use_core=on  pipeline=on  use_rpm=on  gen_core=off
      settings: xl_area=[5 10 0 10 0 0 0]
  a_out : Outport
  bw : Outport  Port=2
  sync_out : Outport  Port=3
  wires:
  convert_im/1 -> ri_to_c/2(im)
  convert_re/1 -> ri_to_c/1(re)
  Delay1/1 -> a_out/1
  a_in/1 -> Delay1/1
  c_to_ri/2(im) -> imim/1, br_add_bi/2
  c_to_ri1/1(re) -> wr_add_wi/1, rere/2
  c_to_ri1/2(im) -> wr_add_wi/2, imim/2
  c_to_ri/1(re) -> rere/1, br_add_bi/1
  Delay/1 -> sync_out/1
  sync_in/1 -> Delay/1
  sumsum/1 -> ss_sub_rrii/1
  ri_to_c/1(c) -> bw/1
  wr_add_wi/1 -> sumsum/2
  br_add_bi/1 -> sumsum/1
  imim/1 -> rr_add_ii/1, rr_sub_ii/2
  rere/1 -> rr_sub_ii/1, rr_add_ii/2
  w/1 -> c_to_ri1/1(c)
  b/1 -> c_to_ri/1(c)
  rr_add_ii/1 -> ss_sub_rrii/2
  rr_sub_ii/1 -> convert_re/1
  ss_sub_rrii/1 -> convert_im/1

== system test_junk/r2_dit_fft/r2_dit_stage_4/r2_twiddle/twiddle_gen1 ==
  sync_in : Inport  Port=1  LatchInput=off
  Counter : xbsIndex_r3/Counter  cnt_type=Free Running  n_bits=9  bin_pt=0  arith_type=Unsigned  start_count=0  cnt_to=Inf  cnt_by_val=1  operation=Up  explicit_period=off  period=1  load_pin=off  rst=on  en=off  dbl_ovrd=off  show_param=off  use_rpm=on  gen_core=off
      settings: xl_area=[0, 0, 0, 0, 0, 0, 0]
  addr_sel : xbsIndex_r3/Slice  mode=Upper Bit Location + Width  nbits=3  bit1=0  base1=MSB of Input  bit0=-1  base0=MSB of Input  boolean_output=off  explicit_period=off  period=1  dbl_ovrd=off
  mem_c : xbsIndex_r3/ROM  depth=8  initVector=[65536;384;47013;215973;60879;237450;25482;202191]  arith_type=Unsigned  n_bits=18  bin_pt=0  latency=1  init_zero=on  explicit_period=off  period=1  rst=off  init_reg=0  en=off  dbl_ovrd=off  show_param=on  distributed_mem=on  use_rpm=on  gen_core=off
      settings: AttributesFormatString=depth = %<depth>\ndist_mem = %<distributed_mem>  xl_area=[0, 0, 0, 0, 0, 0, 0]
  w : Outport
  wires:
  mem_c/1 -> w/1
  addr_sel/1 -> mem_c/1
  Counter/1 -> addr_sel/1
  sync_in/1 -> Counter/1

== system test_junk/r2_dit_fft/r2_dit_stage_5/biplex_commutator/delay_b ==
  in : Inport  Port=1  LatchInput=off
  slr : xbsIndex_r3/Delay  latency=32  reg_retiming=off  explicit_period=off  period=1  en=off  accept_only_valid=off  init_zero=on  dbl_ovrd=off  show_param=off
      settings: xl_area=[0, 0, 0, 0, 0, 0, 0]
  out : Outport
  wires:
  slr/1 -> out/1
  in/1 -> slr/1

== system test_junk/r2_dit_fft/r2_dit_stage_5/biplex_commutator/delay_lo ==
  in : Inport  Port=1  LatchInput=off
  slr : xbsIndex_r3/Delay  latency=32  reg_retiming=off  explicit_period=off  period=1  en=off  accept_only_valid=off  init_zero=on  dbl_ovrd=off  show_param=off
      settings: xl_area=[0, 0, 0, 0, 0, 0, 0]
  out : Outport
  wires:
  slr/1 -> out/1
  in/1 -> slr/1
